simulink model "V4_Modell_EM"  (R2022a)
settings: Solver=ode3  StartTime=0.0  StopTime=Zeit(end)  FixedStep=0.00001  RelTol=1e-3
values from neighbouring files (symbols this model uses):
  k_M = -0.038462    [V4_Parameter_EM.m]    (also in V4_Parameter_Wagen_St.m; V4_Parameter_Wagen_Te.m; V4_Parameter_komplett_St.m; V4_Parameter_komplett_Te.m)
  KL_R_VH = [10      20      30      40 ... (first row only)    [V4_Parameter_EM.m]    (also in V4_Parameter_komplett_St.m; V4_Parameter_komplett_Te.m)
  L_A = 0.11 * (10^(-3))    (= 0.00011)    [V4_Parameter_EM.m]    (also in V4_Parameter_komplett_St.m; V4_Parameter_komplett_Te.m)
  R_A = 0.36    [V4_Parameter_EM.m]    (also in V4_Parameter_komplett_St.m; V4_Parameter_komplett_Te.m)
  r_ZR = 25 * (10^(-3))    (= 0.025)    [V4_Parameter_EM.m]    (also in V4_Parameter_Wagen_St.m = 0.021; V4_Parameter_Wagen_Te.m = 0.021; V4_Parameter_komplett_St.m; V4_Parameter_komplett_Te.m)
settings Model: Creator=bornk  LastModifiedBy=bornk

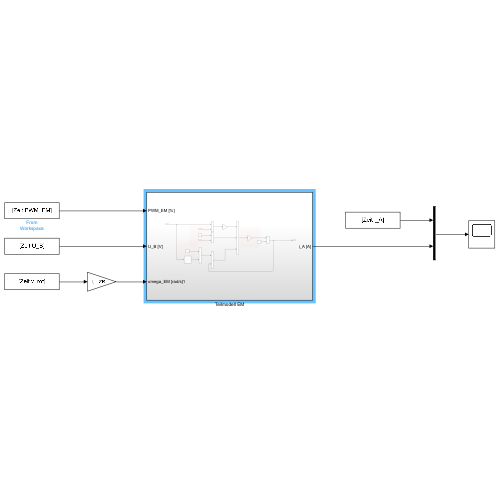
[thumbnail: Simulink's stored preview of the top-level diagram]
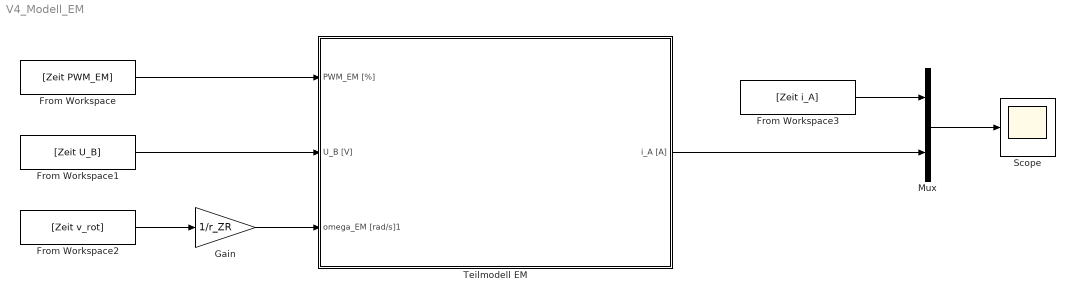
== system V4_Modell_EM ==
  From Workspace : FromWorkspace  VariableName=[Zeit PWM_EM]
  From Workspace1 : FromWorkspace  VariableName=[Zeit U_B]
  From Workspace2 : FromWorkspace  VariableName=[Zeit v_rot]
  From Workspace3 : FromWorkspace  VariableName=[Zeit i_A]
  Gain : Gain  Gain=1/r_ZR
  Mux : Mux  Inputs=2
  Scope : Scope
  Teilmodell EM : Subsystem
  wires:
  From Workspace1/1 -> Teilmodell EM/2(U_B [V])
  From Workspace/1 -> Teilmodell EM/1(PWM_EM [%])
  Gain/1 -> Teilmodell EM/3(omega_EM [rad/s]1)
  From Workspace2/1 -> Gain/1
  From Workspace3/1 -> Mux/1
  Teilmodell EM/1(i_A [A]) -> Mux/2
  Mux/1 -> Scope/1

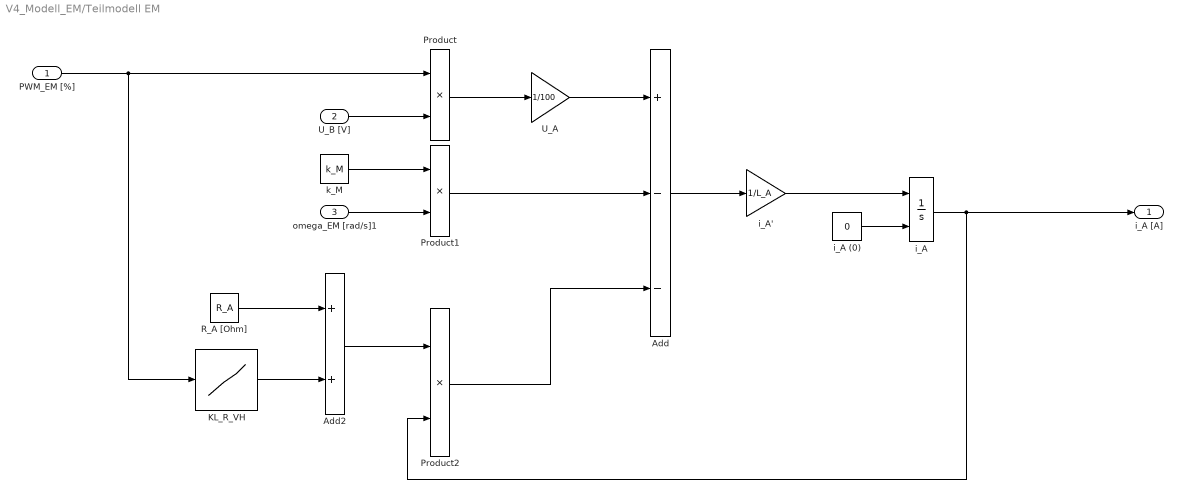
== system V4_Modell_EM/Teilmodell EM ==
  PWM_EM [%] : Inport
  U_B [V] : Inport  Port=2
  omega_EM [rad/s]1 : Inport  Port=3
  Add : Sum  Inputs=+--
  Add2 : Sum
  KL_R_VH : Lookup_n-D  NumberOfTableDimensions=1  BreakpointsForDimension1=KL_R_VH(1,:)  Table=KL_R_VH(2,:)  InternalRulePriority=Speed  RndMeth=Simplest
  Product : Product
  Product1 : Product
  Product2 : Product
  R_A [Ohm] : Constant  Value=R_A
  U_A : Gain  Gain=1/100
  i_A : Integrator  InitialConditionSource=external
  i_A (0) : Constant  Value=0
  i_A' : Gain  Gain=1/L_A
  k_M : Constant  Value=k_M
  i_A [A] : Outport
  wires:
  i_A'/1 -> i_A/1
  i_A (0)/1 -> i_A/2
  i_A/1 -> Product2/2, i_A [A]/1
  Add/1 -> i_A'/1
  Product/1 -> U_A/1
  U_A/1 -> Add/1
  PWM_EM [%]/1 -> KL_R_VH/1, Product/1
  U_B [V]/1 -> Product/2
  Product1/1 -> Add/2
  omega_EM [rad/s]1/1 -> Product1/2
  k_M/1 -> Product1/1
  Product2/1 -> Add/3
  Add2/1 -> Product2/1
  R_A [Ohm]/1 -> Add2/1
  KL_R_VH/1 -> Add2/2
